simulink model "example02_r2022a"  (R2022a)
settings: Solver=VariableStepAuto  StartTime=0.0  StopTime=10.0  RelTol=1e-3
settings Model: Creator=mluser  LastModifiedBy=mluser
settings ModelReferenceCC: EnableRefExpFcnMdlSchedulingChecks=off
settings RTWCC: Description=Generic Real-Time Target

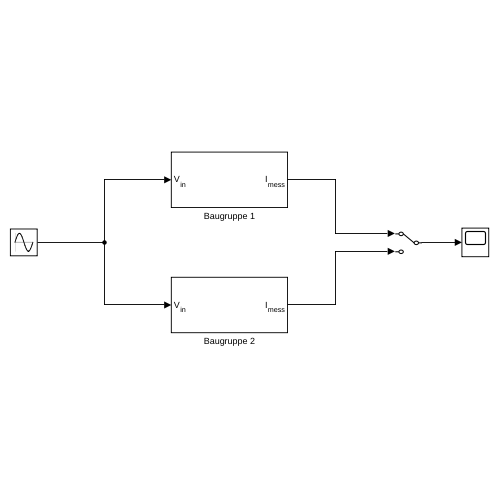
[thumbnail: Simulink's stored preview of the top-level diagram]
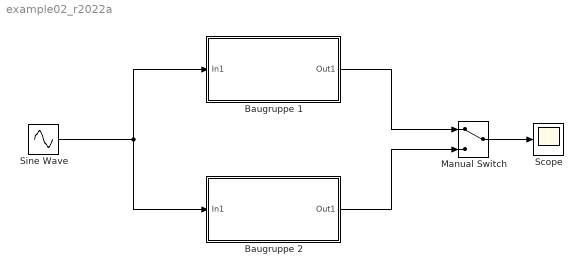
== system example02_r2022a ==
  Baugruppe 1 : Subsystem
      mask Display:
      | port_label('input', 1, 'V_{in}', 'interpreter', 'tex');
      | port_label('output', 1, 'I_{mess}', 'interpreter', 'tex');
  Baugruppe 2 : Subsystem
      mask Display:
      | port_label('input', 1, 'V_{in}', 'interpreter', 'tex');
      | port_label('output', 1, 'I_{mess}', 'interpreter', 'tex');
  Manual Switch : ManualSwitch
  Scope : Scope
  Sine Wave : Sin  SampleTime=0
  wires:
  Sine Wave/1 -> Baugruppe 2/1(In1), Baugruppe 1/1(In1)
  Baugruppe 1/1(Out1) -> Manual Switch/1
  Baugruppe 2/1(Out1) -> Manual Switch/2
  Manual Switch/1 -> Scope/1

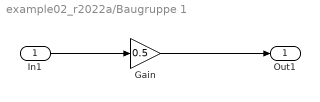
== system example02_r2022a/Baugruppe 1 ==
  In1 : Inport
  Gain : Gain  Gain=0.5
  Out1 : Outport
  wires:
  In1/1 -> Gain/1
  Gain/1 -> Out1/1

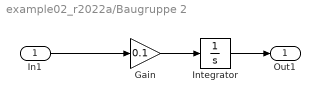
== system example02_r2022a/Baugruppe 2 ==
  In1 : Inport
  Gain : Gain  Gain=0.1
  Integrator : Integrator
  Out1 : Outport
  wires:
  In1/1 -> Gain/1
  Gain/1 -> Integrator/1
  Integrator/1 -> Out1/1
